simulink model "Nominal_Plant"  (R2017a)
settings: Solver=VariableStepAuto  StartTime=0.0  StopTime=10.0  RelTol=1e-3
values from neighbouring files (symbols this model uses):
  A_new = zeros(6,6)    [main_1.m]
  B_new = zeros(6,2)    [main_1.m]
  C_new = [1 0 0 0 0 0;0 1 0 0 0 0;0 0 1 0 0 0]    [main_1.m]
  D_new = zeros(3,2)    [main_1.m]
libraries: cstblocks x9
settings Model: Creator=Ali  LastModifiedBy=Ali
settings DebuggingCC: UnconnectedInputMsg=none  UnconnectedOutputMsg=none  UnconnectedLineMsg=none

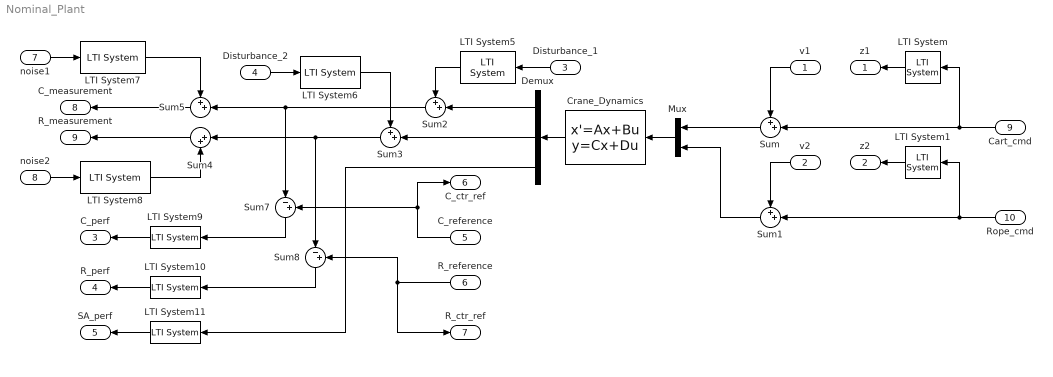
== system Nominal_Plant ==
  v1 : Inport
  v2 : Inport  Port=2
  Disturbance_1 : Inport  Port=3
  Disturbance_2 : Inport  Port=4
  C_reference : Inport  Port=5
  R_reference : Inport  Port=6
  noise1 : Inport  Port=7
  noise2 : Inport  Port=8
  Cart_cmd : Inport  Port=9
  Rope_cmd : Inport  Port=10
  Crane_Dynamics : StateSpace  A=A_new  B=B_new  C=C_new  D=D_new  X0=0
  Demux : Demux  Outputs=3
  LTI System : cstblocks/LTI System  sys=Wa1  IC=[]
  LTI System1 : cstblocks/LTI System  sys=Wa2  IC=[]
  LTI System10 : cstblocks/LTI System  sys=W_L_perf  IC=[]
  LTI System11 : cstblocks/LTI System  sys=W_sa_perf  IC=[]
  LTI System5 : cstblocks/LTI System  sys=W_d_1  IC=[]
  LTI System6 : cstblocks/LTI System  sys=W_d_2  IC=[]
  LTI System7 : cstblocks/LTI System  sys=W_noise1  IC=[]
  LTI System8 : cstblocks/LTI System  sys=W_noise2  IC=[]
  LTI System9 : cstblocks/LTI System  sys=W_P_perf  IC=[]
  Mux : Mux  Inputs=2
  Sum{,1..3,5} (5 alike) : Sum  Inputs=++|
  Sum4 : Sum  Inputs=|++
  Sum7 : Sum  Inputs=|-+
  Sum8 : Sum  Inputs=|-+
  z1 : Outport
  z2 : Outport  Port=2
  C_perf : Outport  Port=3
  R_perf : Outport  Port=4
  SA_perf : Outport  Port=5
  C_ctr_ref : Outport  Port=6
  R_ctr_ref : Outport  Port=7
  C_measurement : Outport  Port=8
  R_measurement : Outport  Port=9
  wires:
  Cart_cmd/1 -> LTI System/1, Sum/2
  LTI System/1 -> z1/1
  LTI System1/1 -> z2/1
  v1/1 -> Sum/1
  v2/1 -> Sum1/1
  Rope_cmd/1 -> LTI System1/1, Sum1/2
  Sum/1 -> Mux/1
  Sum1/1 -> Mux/2
  Mux/1 -> Crane_Dynamics/1
  Crane_Dynamics/1 -> Demux/1
  Demux/1 -> Sum2/2
  Demux/2 -> Sum3/2
  LTI System7/1 -> Sum5/1
  Sum3/1 -> Sum4/1, Sum8/1
  Sum2/1 -> Sum5/2, Sum7/1
  Sum7/1 -> LTI System9/1
  Sum8/1 -> LTI System10/1
  Demux/3 -> LTI System11/1
  C_reference/1 -> C_ctr_ref/1, Sum7/2
  R_reference/1 -> R_ctr_ref/1, Sum8/2
  Disturbance_1/1 -> LTI System5/1
  LTI System5/1 -> Sum2/1
  Disturbance_2/1 -> LTI System6/1
  LTI System6/1 -> Sum3/1
  noise1/1 -> LTI System7/1
  noise2/1 -> LTI System8/1
  LTI System11/1 -> SA_perf/1
  LTI System9/1 -> C_perf/1
  LTI System10/1 -> R_perf/1
  LTI System8/1 -> Sum4/2
  Sum5/1 -> C_measurement/1
  Sum4/1 -> R_measurement/1
